simulink model "AutomaticTransmission"  (R2022b)
settings: Solver=VariableStepAuto  StartTime=0.0  StopTime=50  RelTol=0.001
model workspace (MATLAB code in the model file):
  | load sldemo_autotrans_data; %load initial conditions and other necessary data
values from neighbouring files (symbols this model uses):
  converter_data = [0 0.1 0.2 0.3 0.4 0.5 0.6 0.7 0.8 0.81 0.82 0.83 ... (63 elements, 21x3)]    [hecate_demo_data.mat]
  downtab = [0 0 0 0 0 0 5 5 5 5 30 30 ... (24 elements, 6x4)]    [hecate_demo_data.mat]
  emap = [-40 215 245 264 264 267 267 267 267 267 -44 117 ... (110 elements, 10x11)]    [hecate_demo_data.mat]
  Iei = 0.0219914882836    [hecate_demo_data.mat]
  uptab = [10 10 15 23 40 40 30 30 30 41 70 70 ... (24 elements, 6x4)]    [hecate_demo_data.mat]
  vehicledata = [3.23 40 0.02 1 12.0941478573 0]    [hecate_demo_data.mat]
undefined symbols (not defined in the file or in its folder): Hecate_brakeAmp, Hecate_brakePeriod, Hecate_throttle, Hecate_throttleDuration, Hecate_throttleMax, Hecate_throttleSlope
settings Model: DataTypeOverride=Off  MinMaxOverflowLogging=ForceOff  SimulationMode=accelerator  LastModifiedBy=fedformi_new
settings SolverCC: ConsecutiveZCsStepRelTol=2.8421709430404e-13
settings DataIOCC: SaveFormat=Array
settings OptimizationCC: BlockReduction=off  BooleanDataType=off
settings DebuggingCC: SaveWithParameterizedLinksMsg=none  UnderspecifiedInitializationDetection=Classic  MergeDetectMultiDrivingBlocksExec=none  SignalResolutionControl=TryResolveAllWithWarning
settings HardwareCC: TargetUnknown=on
settings ModelReferenceCC: PropagateSignalLabelsOutOfModel=off

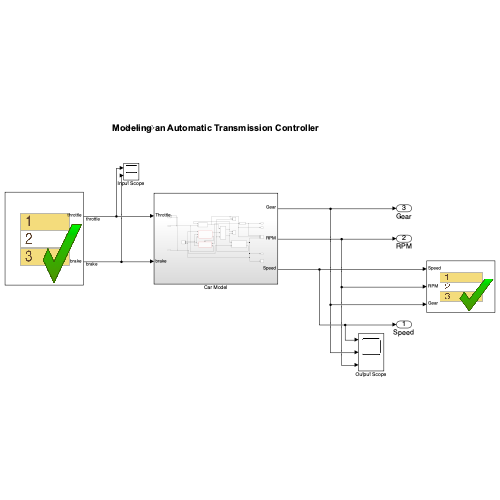
[thumbnail: Simulink's stored preview of the top-level diagram]
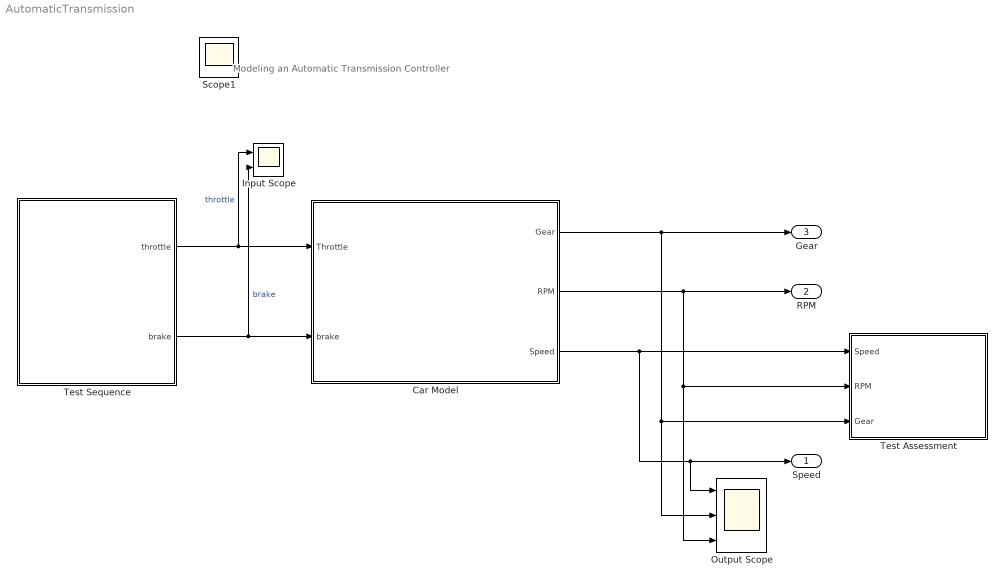
== system AutomaticTransmission ==
  note: Modeling an Automatic Transmission Controller
  Car Model : Subsystem
  Input Scope : Scope  NumInputPorts=2
  Output Scope : Scope  NumInputPorts=3
  Test Assessment : Test Sequence  TreatAsAtomicUnit=on
  Test Sequence : Test Sequence  TreatAsAtomicUnit=on
  Speed : Outport  VectorParamsAs1DForOutWhenUnconnected=off
  RPM : Outport  Port=2  VectorParamsAs1DForOutWhenUnconnected=off
  Gear : Outport  Port=3  VectorParamsAs1DForOutWhenUnconnected=off
  Scope1 : Scope
  wires:
  Test Sequence/1(throttle) -> Input Scope/1, Car Model/1(Throttle)  "throttle"
  Test Sequence/2(brake) -> Input Scope/2, Car Model/2(brake)  "brake"
  Car Model/3(Speed) -> Test Assessment/1(Speed), Output Scope/1, Speed/1
  Car Model/2(RPM) -> RPM/1, Output Scope/3, Test Assessment/2(RPM)
  Car Model/1(Gear) -> Test Assessment/3(Gear), Output Scope/2, Gear/1
  ? -> ?

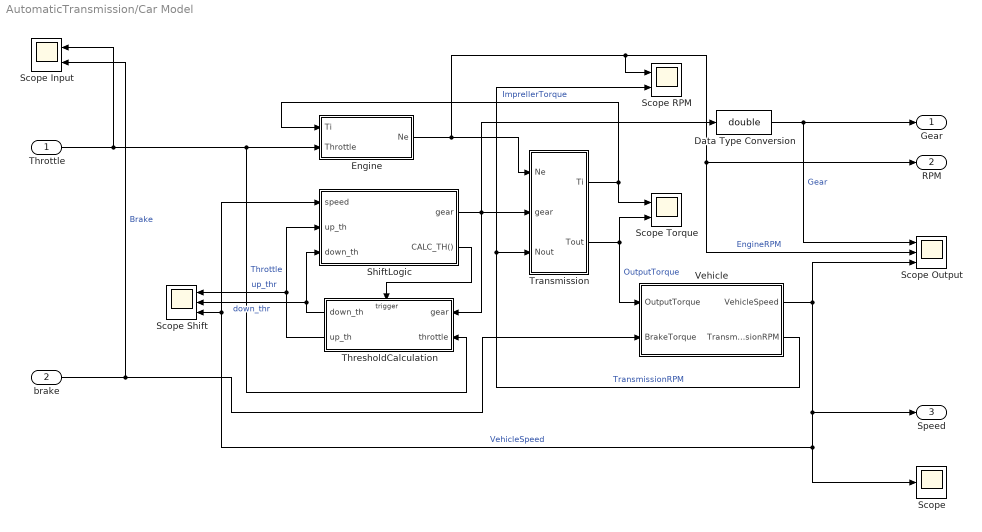
== system AutomaticTransmission/Car Model ==
  Throttle : Inport
  brake : Inport  Port=2
  Data Type Conversion : DataTypeConversion  OutDataTypeStr=double  SaturateOnIntegerOverflow=off  RndMeth=Floor
  Engine : Subsystem
  Scope : Scope
  Scope Input : Scope  NumInputPorts=2
  Scope Output : Scope  NumInputPorts=3
  Scope RPM : Scope  NumInputPorts=2
  Scope Shift : Scope  NumInputPorts=3
  Scope Torque : Scope  NumInputPorts=2
  ShiftLogic : Stateflow chart  TreatAsAtomicUnit=on
  ThresholdCalculation : Subsystem  TreatAsAtomicUnit=on
  Transmission : Subsystem
  Vehicle : Subsystem  mask(vehicle model){Rfd=vehicledata(1), rload0=vehicledata(2), rload2=vehicledata(3), Rw=vehicledata(4), Iv=vehicledata(5), N20=vehicledata(6)/vehicledata(4)*vehicledata(1)}
      mask prompts: Rfd "final drive ratio"; rload0 "drag friction at wheels"; rload2 "aerodynamic drag"; Rw "wheel radius"; Iv "vehicle inertia"; N20 "initial transmission output speed"
      mask help: vehicle dynamics: torque input from trans., outputs are input speed (transmission output) and vehicle speed
      mask Display: image(imread([matlabroot,'/toolbox/simulink/simdemos/automotive/html/NSX_3Colors.jpg']))
  Gear : Outport  VectorParamsAs1DForOutWhenUnconnected=off
  RPM : Outport  Port=2  VectorParamsAs1DForOutWhenUnconnected=off
  Speed : Outport  Port=3  VectorParamsAs1DForOutWhenUnconnected=off
  wires:
  Throttle/1 -> Engine/2(Throttle), ThresholdCalculation/2(throttle), Scope Input/1  "Throttle"
  Engine/1(Ne) -> Transmission/1(Ne), Scope RPM/1, RPM/1, Scope Output/2  "EngineRPM"
  Vehicle/2(TransmissionRPM) -> Transmission/3(Nout), Scope RPM/2  "TransmissionRPM"
  ThresholdCalculation/2(up_th) -> ShiftLogic/2(up_th), Scope Shift/1  "up_thr"
  brake/1 -> Vehicle/2(BrakeTorque), Scope Input/2  "Brake"
  Vehicle/1(VehicleSpeed) -> Scope/1, Scope Shift/3, ShiftLogic/1(speed), Speed/1, Scope Output/3  "VehicleSpeed"
  Transmission/1(Ti) -> Engine/1(Ti), Scope Torque/1  "ImprellerTorque"
  ShiftLogic/2(CALC_TH()) -> ThresholdCalculation/Trigger
  ShiftLogic/1(gear) -> Transmission/2(gear), ThresholdCalculation/1(gear), Data Type Conversion/1
  Transmission/2(Tout) -> Vehicle/1(OutputTorque), Scope Torque/2  "OutputTorque"
  ThresholdCalculation/1(down_th) -> Scope Shift/2, ShiftLogic/3(down_th)  "down_thr"
  Data Type Conversion/1 -> Gear/1, Scope Output/1  "Gear"

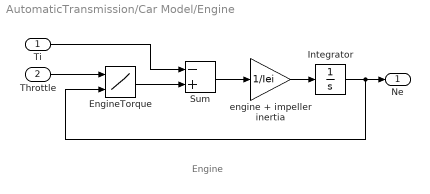
== system AutomaticTransmission/Car Model/Engine ==
  note: Engine
  Ti : Inport
  Throttle : Inport  Port=2
  EngineTorque : Lookup2D  RowIndex=thvec  ColumnIndex=nevec  Table=emap  SaturateOnIntegerOverflow=off
  Integrator : Integrator  InitialCondition=1000  LimitOutput=on  UpperSaturationLimit=6000  LowerSaturationLimit=600  ZeroCross=off
  Sum : Sum  Inputs=-+  InputSameDT=on  SaturateOnIntegerOverflow=on  OutDataTypeStr=Inherit: Same as first input
  engine + impeller inertia : Gain  Gain=1/Iei  SaturateOnIntegerOverflow=on  OutDataTypeStr=Inherit: Same as input  ParamDataTypeStr=Inherit: Same as input
  Ne : Outport  InitialOutput=0  VectorParamsAs1DForOutWhenUnconnected=off
  wires:
  Ti/1 -> Sum/1
  Throttle/1 -> EngineTorque/1
  Integrator/1 -> EngineTorque/2, Ne/1
  Sum/1 -> engine + impeller inertia/1
  engine + impeller inertia/1 -> Integrator/1
  EngineTorque/1 -> Sum/2

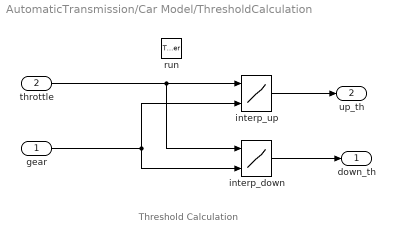
== system AutomaticTransmission/Car Model/ThresholdCalculation ==
  note: Threshold Calculation
  gear : Inport
  throttle : Inport  Port=2
  run : TriggerPort  TriggerType=function-call  VariantControl=(inherit)  ZeroCross=off
  interp_down : Lookup2D  RowIndex=downth  ColumnIndex=[1:4]  Table=downtab  OutDataTypeStr=double  SaturateOnIntegerOverflow=off  InputSameDT=off
      settings: LockScale=on
  interp_up : Lookup2D  RowIndex=upth  ColumnIndex=[1:4]  Table=uptab  OutDataTypeStr=double  SaturateOnIntegerOverflow=off  InputSameDT=off
      settings: LockScale=on
  down_th : Outport  VectorParamsAs1DForOutWhenUnconnected=off
  up_th : Outport  Port=2  VectorParamsAs1DForOutWhenUnconnected=off
  wires:
  interp_up/1 -> up_th/1
  interp_down/1 -> down_th/1
  throttle/1 -> interp_up/1, interp_down/1
  gear/1 -> interp_up/2, interp_down/2

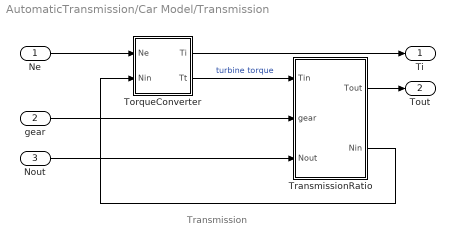
== system AutomaticTransmission/Car Model/Transmission ==
  note: Transmission
  Ne : Inport
  gear : Inport  Port=2
  Nout : Inport  Port=3
  TorqueConverter : Subsystem  mask(torque converter){speedratio=converter_data(:,1), Kfactor=converter_data(:,2), Torkratio=converter_data(:,3)}
      mask prompts: speedratio "speed ratio"; Kfactor "K factor"; Torkratio "torque ratio"
      mask help: torque converter
      mask Help: Torque converter input and output torques are computed as a function of the input and output speeds
      mask Display: plot([cos([90:10:450]*pi/180),.63*cos([90:10:450]*pi/180),.63*cos([90:10:240]*pi/180),cos([240:10:300]*pi/180),.63*cos([300]*pi/180)],[sin([90:10:450]*pi/180),.63*sin([90:10:450]*pi/180)+.1,.63*sin([90:10:240]*pi/180)+.1,sin([240:10:300]*pi/180),.63*sin([300]*pi/180)+.1])
  TransmissionRatio : Subsystem
  Ti : Outport  InitialOutput=0  VectorParamsAs1DForOutWhenUnconnected=off
  Tout : Outport  Port=2  InitialOutput=0  VectorParamsAs1DForOutWhenUnconnected=off
  wires:
  TransmissionRatio/1(Tout) -> Tout/1
  TorqueConverter/1(Ti) -> Ti/1
  Nout/1 -> TransmissionRatio/3(Nout)
  gear/1 -> TransmissionRatio/2(gear)
  Ne/1 -> TorqueConverter/1(Ne)
  TransmissionRatio/2(Nin) -> TorqueConverter/2(Nin)
  TorqueConverter/2(Tt) -> TransmissionRatio/1(Tin)  "turbine torque"

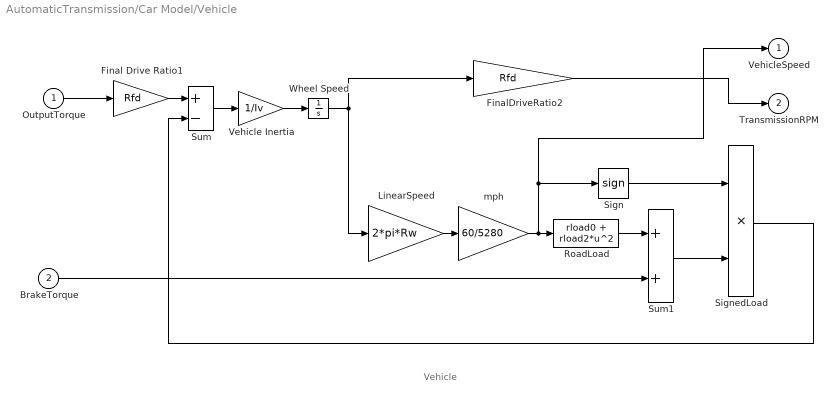
== system AutomaticTransmission/Car Model/Vehicle ==
  note: Vehicle
  OutputTorque : Inport
  BrakeTorque : Inport  Port=2
  Final Drive Ratio1 : Gain  Gain=Rfd  SaturateOnIntegerOverflow=on  OutDataTypeStr=Inherit: Same as input  ParamDataTypeStr=Inherit: Same as input
  FinalDriveRatio2 : Gain  Gain=Rfd  SaturateOnIntegerOverflow=on  OutDataTypeStr=Inherit: Same as input  ParamDataTypeStr=Inherit: Same as input
  LinearSpeed : Gain  Gain=2*pi*Rw  SaturateOnIntegerOverflow=on  OutDataTypeStr=Inherit: Same as input  ParamDataTypeStr=Inherit: Same as input
  RoadLoad : Fcn  Expr=rload0 + rload2*u^2
  Sign : Signum
  SignedLoad : Product  InputSameDT=on  SaturateOnIntegerOverflow=on  OutDataTypeStr=Inherit: Same as first input
  Sum : Sum  Inputs=+-  InputSameDT=on  SaturateOnIntegerOverflow=on  OutDataTypeStr=Inherit: Same as first input
  Sum1 : Sum  InputSameDT=on  SaturateOnIntegerOverflow=on  OutDataTypeStr=Inherit: Same as first input
  Vehicle Inertia : Gain  Gain=1/Iv  SaturateOnIntegerOverflow=on  OutDataTypeStr=Inherit: Same as input  ParamDataTypeStr=Inherit: Same as input
  Wheel Speed : Integrator  InitialCondition=N20/Rfd  ZeroCross=off
  mph : Gain  Gain=60/5280  SaturateOnIntegerOverflow=on  OutDataTypeStr=Inherit: Same as input  ParamDataTypeStr=Inherit: Same as input
  VehicleSpeed : Outport  InitialOutput=0  VectorParamsAs1DForOutWhenUnconnected=off
  TransmissionRPM : Outport  Port=2  InitialOutput=0  VectorParamsAs1DForOutWhenUnconnected=off
  wires:
  FinalDriveRatio2/1 -> TransmissionRPM/1
  BrakeTorque/1 -> Sum1/2
  Sum1/1 -> SignedLoad/2
  RoadLoad/1 -> Sum1/1
  Sign/1 -> SignedLoad/1
  SignedLoad/1 -> Sum/2
  OutputTorque/1 -> Final Drive Ratio1/1
  Vehicle Inertia/1 -> Wheel Speed/1
  Sum/1 -> Vehicle Inertia/1
  mph/1 -> VehicleSpeed/1, Sign/1, RoadLoad/1
  LinearSpeed/1 -> mph/1
  Wheel Speed/1 -> LinearSpeed/1, FinalDriveRatio2/1
  Final Drive Ratio1/1 -> Sum/1

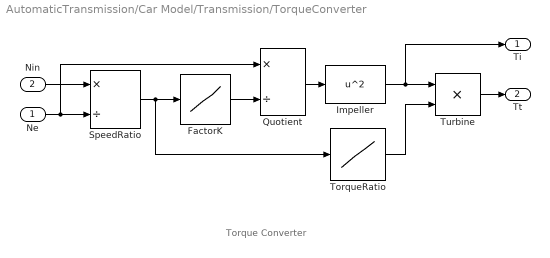
== system AutomaticTransmission/Car Model/Transmission/TorqueConverter ==
  note: Torque Converter
  Ne : Inport
  Nin : Inport  Port=2
  FactorK : Lookup  InputValues=speedratio  Table=Kfactor
  Impeller : Fcn  Expr=u^2
  Quotient : Product  Inputs=*/  InputSameDT=on  SaturateOnIntegerOverflow=on  OutDataTypeStr=Inherit: Same as first input
  SpeedRatio : Product  Inputs=*/  InputSameDT=on  SaturateOnIntegerOverflow=on  OutDataTypeStr=Inherit: Same as first input
  TorqueRatio : Lookup  InputValues=speedratio  Table=Torkratio
  Turbine : Product  InputSameDT=on  SaturateOnIntegerOverflow=on  OutDataTypeStr=Inherit: Same as first input
  Ti : Outport  InitialOutput=0  VectorParamsAs1DForOutWhenUnconnected=off
  Tt : Outport  Port=2  InitialOutput=0  VectorParamsAs1DForOutWhenUnconnected=off
  wires:
  TorqueRatio/1 -> Turbine/2
  Quotient/1 -> Impeller/1
  FactorK/1 -> Quotient/2
  SpeedRatio/1 -> TorqueRatio/1, FactorK/1
  Impeller/1 -> Turbine/1, Ti/1
  Turbine/1 -> Tt/1
  Ne/1 -> SpeedRatio/2, Quotient/1
  Nin/1 -> SpeedRatio/1

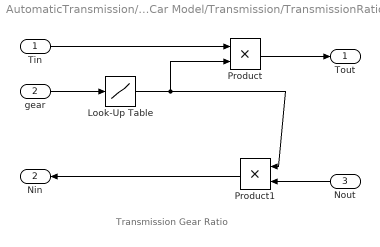
== system AutomaticTransmission/Car Model/Transmission/TransmissionRatio ==
  note: Transmission Gear Ratio
  Tin : Inport
  gear : Inport  Port=2
  Nout : Inport  Port=3
  Look-Up Table : Lookup  InputValues=[1 2 3 4]  Table=[2.393 1.450 1.000 0.677]  OutDataTypeStr=double  LockScale=on
  Product : Product  InputSameDT=on  SaturateOnIntegerOverflow=on  OutDataTypeStr=Inherit: Same as first input
  Product1 : Product  InputSameDT=on  SaturateOnIntegerOverflow=on  OutDataTypeStr=Inherit: Same as first input
  Tout : Outport  InitialOutput=0  VectorParamsAs1DForOutWhenUnconnected=off
  Nin : Outport  Port=2  InitialOutput=0  VectorParamsAs1DForOutWhenUnconnected=off
  wires:
  Look-Up Table/1 -> Product1/1, Product/2
  Nout/1 -> Product1/2
  Product1/1 -> Nin/1
  Product/1 -> Tout/1
  Tin/1 -> Product/1
  gear/1 -> Look-Up Table/1

== stateflow chart AutomaticTransmission/Test Sequence ==
  state Manual
    state step_1
      throttle = 50;
      brake = 0;
    state step_2
      throttle = 10;
      brake = 20;
    state step_3
      throttle = 70;
      brake = 0;
      settings: description=|
          | Throttle = 70: Fail
          | Throttle = 60: Pass
    (default) -> Manual.step_1
    Manual.step_1 -> Manual.step_2 : [
        | et > 30
        | ]
    Manual.step_2 -> Manual.step_3 : [
        | et > 5
        | ]
  state ThreeSteps
    state step_1
      throttle = 50;
      brake = 0;
    state step_2
      throttle = 10;
      brake = 20;
    state step_3
      throttle = Hecate_throttle;
      brake = 0;
      settings: description=|
          | Throttle = 70: Fail
          | Throttle = 60: Pass
    (default) -> ThreeSteps.step_1
    ThreeSteps.step_1 -> ThreeSteps.step_2 : [
        | et > 30
        | ]
    ThreeSteps.step_2 -> ThreeSteps.step_3 : [
        | et > 5
        | ]
  state Trapezoidal
    state Brake
      brake = Hecate_brakeAmp + Hecate_brakeAmp*sin(2*pi/Hecate_brakePeriod*t);
      state RisingThrottle
        throttle = Hecate_throttleMax*0.1*t;
      state ConstantThrottle
        throttle = Hecate_throttleMax;
      state LoweringThrottle
        throttle = Hecate_throttleMax*(1-et*Hecate_throttleSlope);
      state SinkState
        throttle = 0;
      (default) -> RisingThrottle
      RisingThrottle -> ConstantThrottle : [
          | t >= 10
          | ]
      ConstantThrottle -> LoweringThrottle : [
          | et >= Hecate_throttleDuration
          | ]
      LoweringThrottle -> SinkState : [
          | throttle <= 0
          | ]
    (default) -> Brake
  (default) -> Manual [order 1] : [Active_Scenario_Index == 1]
  (default) -> ThreeSteps [order 2] : [Active_Scenario_Index == 2]
  (default) -> Trapezoidal [order 3] : {assert(Active_Scenario_Index == 3,'The value of Scenario Parameter ''Active_Scenario_Index'' is not valid. Use the index of the scenario to specify it.')}
  data: throttle output; brake output; Active_Scenario_Index parameter =2; Hecate_throttle parameter; Hecate_brakeAmp parameter; Hecate_brakePeriod parameter; Hecate_throttleMax parameter; Hecate_throttleDuration parameter; Hecate_throttleSlope parameter

== stateflow chart AutomaticTransmission/Car Model/ShiftLogic ==
  settings: updateMethod=DISCRETE  sampleTime=0.04
  state gear_state [parallel]
    settings: executionOrder=1
    state fourth
      entry:
      gear = 4;
    state third
      entry:
      gear = 3;
    state second
      entry:
      gear = 2;
    state first
      entry:
      gear = 1;
    (default) -> first
    second -> third [order 1] : UP
    first -> second : UP
    third -> fourth [order 1] : UP
    second -> first [order 2] : DOWN
    fourth -> third : DOWN
    third -> second [order 2] : DOWN
  state selection_state [parallel]
    during: CALC_TH;
    settings: executionOrder=2
    state steady_state
    state upshifting
    state downshifting
    (default) -> steady_state
    steady_state -> upshifting [order 1] : [speed > up_th]
    steady_state -> downshifting [order 2] : [speed < down_th]
    downshifting -> steady_state [order 1] : after(TWAIT,tick)
        | [speed <= down_th]
        | {gear_state.DOWN}
    downshifting -> steady_state [order 2] : [speed > down_th]
    upshifting -> steady_state [order 1] : after(TWAIT,tick)
        | [speed >= up_th]
        | {gear_state.UP}
    upshifting -> steady_state [order 2] : [speed < up_th]
  data: speed input double; gear output fixdt(0,8,5) [1..4]; TWAIT parameter fixdt(0,8,6); up_th input double; down_th input double
  events: DOWN local EITHER_EDGE_EVENT; UP local EITHER_EDGE_EVENT; CALC_TH output FUNCTION_CALL_EVENT

== stateflow chart AutomaticTransmission/Test Assessment ==
  state SpeedLimit
    state step_1
      verify(Speed <= 120)
    (default) -> step_1
  state TestGear
    state ParentState
      % Check nothing
      state WaitForGear4
        % Check nothing
      state Pause
        % Check nothing
      state SpeedCheck
        verify(Speed <= 115);
      (default) -> WaitForGear4
      (junction 898) -> WaitForGear4
      (junction 900) -> (junction 898)
      WaitForGear4 -> Pause : [
          | Gear == 4
          | ]
      Pause -> WaitForGear4 [order 1] : [
          | Gear < 4
          | ]
      Pause -> SpeedCheck [order 2] : [
          | et >= 5
          | ]
      SpeedCheck -> (junction 900) : [
          | Gear < 4
          | ]
    state SinkState
      % Check nothing
    (default) -> ParentState
    ParentState -> SinkState : [
        | t >= 25
        | ]
  (default) -> SpeedLimit [order 1] : [Active_Scenario_Index == 1]
  (default) -> TestGear [order 2] : {assert(Active_Scenario_Index == 2,'The value of Scenario Parameter ''Active_Scenario_Index'' is not valid. Use the index of the scenario to specify it.')}
  data: Speed input; RPM input; Gear input; Active_Scenario_Index parameter =1
